simulink model "task_1_x1(t)"  (R2020b)
settings: Solver=VariableStepAuto  StartTime=0.0  StopTime=3.0  RelTol=1e-3
values from neighbouring files (symbols this model uses):
  A = [1, -2, 3; 2, -3, 2; -2, 1, -4]    [task_1.m]    (also in task_2.m; task_3.m = [-8, -3, -12; -3, -2, -6; 6, 0, 7]; task_4.m = [-8, -3, -12; -3, -2, -6; 6, 0, 7])
  B = [-3; -1; 3]    [task_1.m]    (also in task_2.m = [3; 1; -1]; task_3.m = [0; 0; 0]; task_4.m = [0; 0; 0])
settings Model: Creator=dkravchenko  LastModifiedBy=vital

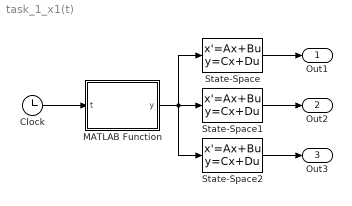
== system task_1_x1(t) ==
  Clock : Clock
  MATLAB Function : MATLAB Function  TreatAsAtomicUnit=on
  State-Space : StateSpace  A=A  B=B  C=[1, 0, 0]  D=0  InitialCondition=0
  State-Space1 : StateSpace  A=A  B=B  C=[0, 1, 0]  D=0  InitialCondition=0
  State-Space2 : StateSpace  A=A  B=B  C=[0, 0, 1]  D=0  InitialCondition=0
  Out1 : Outport
  Out2 : Outport  Port=2
  Out3 : Outport  Port=3
  wires:
  Clock/1 -> MATLAB Function/1(t)
  State-Space/1 -> Out1/1
  State-Space1/1 -> Out2/1
  State-Space2/1 -> Out3/1
  MATLAB Function/1(y) -> State-Space2/1, State-Space/1, State-Space1/1

== matlab function task_1_x1(t)/MATLAB Function ==
  data: t input; y output
function y = u(t)

A = [1, -2, 3; 2, -3, 2; -2, 1, -4];
 
B = [-3; -1; 3];

x_1 = [4; 3; -3];

Gr_t_1 =     [0.7991,    0.2127,   -0.9056;
    0.2127,    0.0612,   -0.2350;
   -0.9056,   -0.2350,    1.0345];

y = B'*expm(A'*(3-t))*inv(Gr_t_1)*x_1;
